simulink model "Prvi2012B"  (R2012b)
settings: Solver=ode45  SolverMode=SingleTasking  StartTime=0.0  StopTime=100  RelTol=1e-3
settings Model: CovMetricSettings=dwe  CovHtmlReporting=off  covSaveCumulativeToWorkspaceVar=off  CovSaveSingleToWorkspaceVar=off  CovExternalEMLEnable=on  Creator=Aldin  LastModifiedBy=Aldin
settings DataIOCC: LimitDataPoints=off  SaveFormat=StructureWithTime  ReturnWorkspaceOutputs=on
settings OptimizationCC: ExpressionDepthLimit=128
settings DebuggingCC: UnderspecifiedInitializationDetection=Simplified  MergeDetectMultiDrivingBlocksExec=error  SolverPrmCheckMsg=none  FrameProcessingCompatibilityMsg=error  StateNameClashWarn=none  SFUnexpectedBacktrackingDiag=error  SFNoUnconditionalDefaultTransitionDiag=error
settings HardwareCC: ProdBitPerPointer=64  ProdLargestAtomicFloat=Float  ProdIntDivRoundTo=Zero  ProdEndianess=LittleEndian  ProdHWDeviceType=Specified
settings ModelReferenceCC: PropagateSignalLabelsOutOfModel=on
settings SFSimCC: SimUseLocalCustomCode=on
settings RTWCC: RTWUseLocalCustomCode=on
settings CodeAppCC: CustomSymbolStrType=$N$R$M_T
settings GRTTargetCC: CodeReplacementLibrary=C99 (ISO)

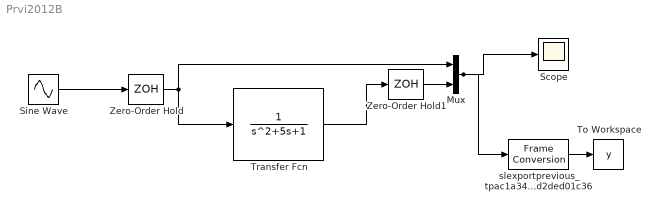
== system Prvi2012B ==
  Mux : Mux  Inputs=2
  Scope : Scope
      settings: TimeRange=auto  MaxDataPoints=5000  SaveToWorkspace=off  SaveName=ScopeData  YMin=-4.99996  YMax=4.99996  SampleTime=-1
  Sine Wave : Sin  Amplitude=4  Frequency=0.25  SampleTime=0.1
  To Workspace : ToWorkspace  VariableName=y  SampleTime=-1
  Transfer Fcn : TransferFcn  Denominator=[1 5 1]
  Zero-Order Hold : ZeroOrderHold  SampleTime=0.1
  Zero-Order Hold1 : ZeroOrderHold  SampleTime=0.1
  slexportprevious_tpac1a347c_b890_4d2e_b2d6_f8d2ded01c36 : FrameConversion  OutFrame=Sample-based
  wires:
  Zero-Order Hold/1 -> Mux/1, Transfer Fcn/1
  Mux/1 -> Scope/1, slexportprevious_tpac1a347c_b890_4d2e_b2d6_f8d2ded01c36/1
  Zero-Order Hold1/1 -> Mux/2
  Transfer Fcn/1 -> Zero-Order Hold1/1
  Sine Wave/1 -> Zero-Order Hold/1
  slexportprevious_tpac1a347c_b890_4d2e_b2d6_f8d2ded01c36/1 -> To Workspace/1
